simulink model "dadtetest"  (R2024a)
settings: Solver=VariableStepAuto  StartTime=0.0  StopTime=1  RelTol=1e-3
libraries: simulink x1
settings Model: Creator=wsl  LastModifiedBy=wsl

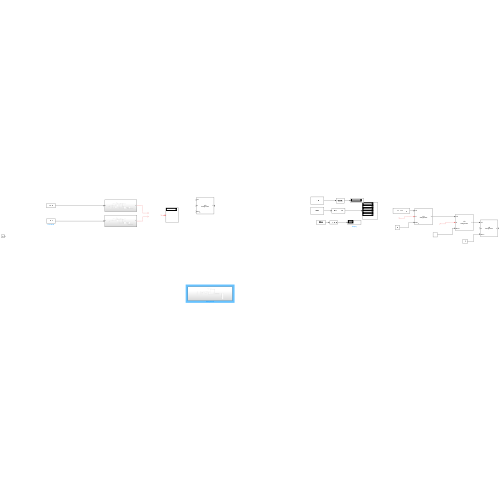
[thumbnail: Simulink's stored preview of the top-level diagram]
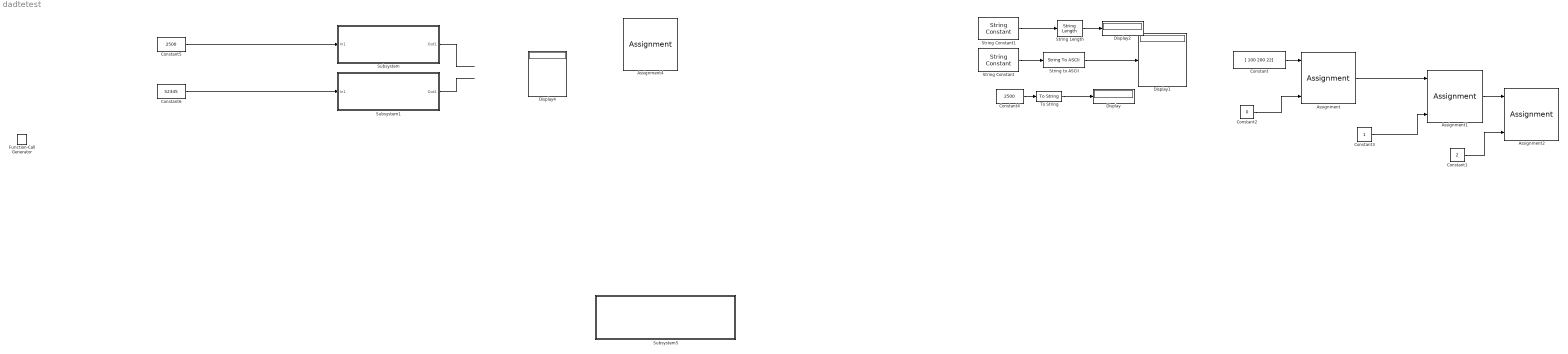
== system dadtetest ==
  Assignment : Assignment  IndexMode=Zero-based  DiagnosticForDimensions=Warning  IndexOptions=Index vector (port)  Indices=2  OutputSizes=1
  Assignment1 : Assignment  IndexMode=Zero-based  DiagnosticForDimensions=Warning  IndexOptions=Index vector (port)  Indices=2  OutputSizes=1
  Assignment2 : Assignment  IndexMode=Zero-based  DiagnosticForDimensions=Warning  IndexOptions=Index vector (port)  Indices=2  OutputSizes=1
  Assignment4 : Assignment  NumberOfDimensions=2  IndexMode=Zero-based  DiagnosticForDimensions=Warning  IndexOptions=Index vector (port),Index vector (dialog)  Indices=2,1  OutputSizes=1,1
  Constant : Constant  Value=[ 100 200 22]  OutDataTypeStr=single
  Constant1 : Constant  Value=2  OutDataTypeStr=uint8
  Constant2 : Constant  Value=0  OutDataTypeStr=uint8
  Constant3 : Constant  OutDataTypeStr=uint8
  Constant4 : Constant  Value=2500  OutDataTypeStr=uint16
  Constant5 : Constant  Value=2500  OutDataTypeStr=uint16
  Constant6 : Constant  Value=52345  OutDataTypeStr=uint16
  Display{,1..2,4} (4 alike) : Display
  Function-Call Generator : simulink/Ports & Subsystems/Function-Call Generator  sample_time=0.01  numberOfIterations=1  DisallowWideOutput=off
  String Constant : StringConstant  String='65535'
  String Constant1 : StringConstant  String='1234'
  String Length : StringLength  OutDataTypeStr=uint8
  String to ASCII : StringToASCII  OutputVectorSize=5
  Subsystem : Subsystem
  Subsystem1 : Subsystem
  Subsystem5 : Subsystem
  To String : ToString
  wires:
  Constant/1 -> Assignment/1
  ? -> Assignment/2
  Constant2/1 -> Assignment/3
  Assignment/1 -> Assignment1/1
  ? -> Assignment1/2
  Constant3/1 -> Assignment1/3
  Assignment1/1 -> Assignment2/1
  Constant1/1 -> Assignment2/3
  Constant4/1 -> To String/1
  To String/1 -> Display/1
  String to ASCII/1 -> Display1/1
  String Constant/1 -> String to ASCII/1
  String Length/1 -> Display2/1
  String Constant1/1 -> String Length/1
  Constant5/1 -> Subsystem/1(In1)
  Constant6/1 -> Subsystem1/1(In1)
  Subsystem/1(Out1) -> ?
  Subsystem1/1(Out1) -> ?
  ? -> Display4/1

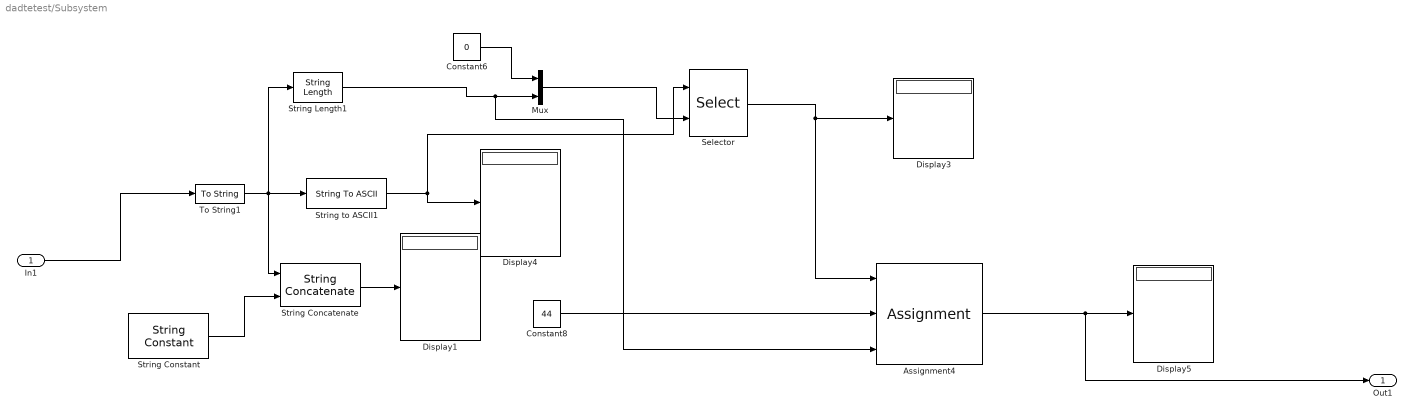
== system dadtetest/Subsystem ==
  In1 : Inport
  Assignment4 : Assignment  IndexMode=Zero-based  DiagnosticForDimensions=Warning  IndexOptions=Index vector (port)  Indices=2  OutputSizes=1
  Constant6 : Constant  Value=0  OutDataTypeStr=uint8
  Constant8 : Constant  Value=44  OutDataTypeStr=uint8
  Display{1,3..5} (4 alike) : Display
  Mux : Mux  Inputs=2
  Selector : Selector  IndexMode=Zero-based  InputPortWidth=6  IndexOptions=Starting and ending indices (port)  Indices=[1 3]  OutputSizes=1
  String Concatenate : StringConcatenate
  String Constant : StringConstant  String="\",\""
  String Length1 : StringLength  OutDataTypeStr=uint8
  String to ASCII1 : StringToASCII  OutputVectorSize=6
  To String1 : ToString
  Out1 : Outport
  wires:
  In1/1 -> To String1/1
  String Length1/1 -> Assignment4/3, Mux/2
  Constant6/1 -> Mux/1
  Constant8/1 -> Assignment4/2
  String to ASCII1/1 -> Selector/1, Display4/1
  Selector/1 -> Assignment4/1, Display3/1
  Mux/1 -> Selector/2
  Assignment4/1 -> Out1/1, Display5/1
  To String1/1 -> String Concatenate/1, String Length1/1, String to ASCII1/1
  String Constant/1 -> String Concatenate/2
  String Concatenate/1 -> Display1/1

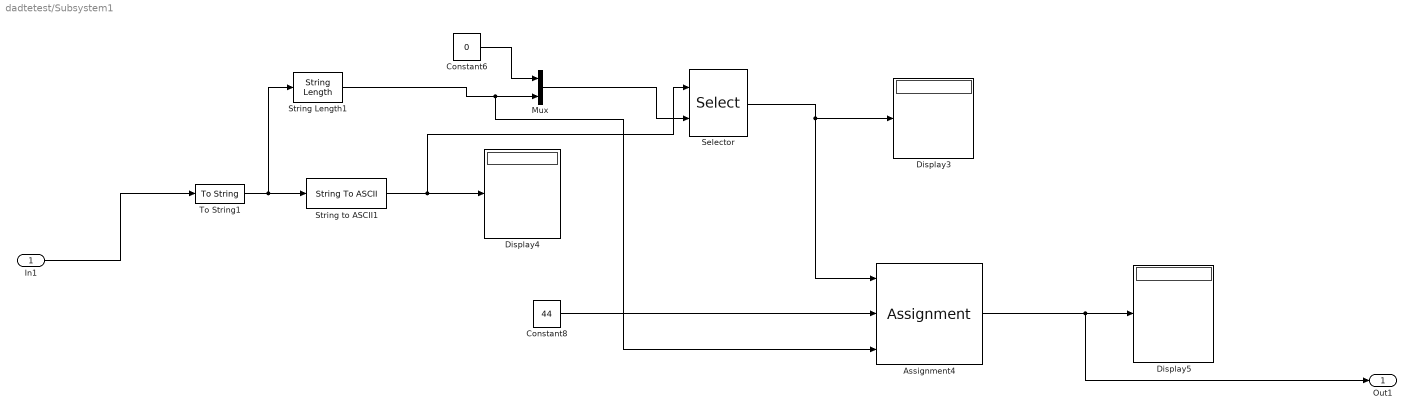
== system dadtetest/Subsystem1 ==
  In1 : Inport
  Assignment4 : Assignment  IndexMode=Zero-based  DiagnosticForDimensions=Warning  IndexOptions=Index vector (port)  Indices=2  OutputSizes=1
  Constant6 : Constant  Value=0  OutDataTypeStr=uint8
  Constant8 : Constant  Value=44  OutDataTypeStr=uint8
  Display3 : Display
  Display4 : Display
  Display5 : Display
  Mux : Mux  Inputs=2
  Selector : Selector  IndexMode=Zero-based  InputPortWidth=6  IndexOptions=Starting and ending indices (port)  Indices=[1 3]  OutputSizes=1
  String Length1 : StringLength  OutDataTypeStr=uint8
  String to ASCII1 : StringToASCII  OutputVectorSize=6
  To String1 : ToString
  Out1 : Outport
  wires:
  In1/1 -> To String1/1
  String Length1/1 -> Assignment4/3, Mux/2
  Constant6/1 -> Mux/1
  Constant8/1 -> Assignment4/2
  String to ASCII1/1 -> Selector/1, Display4/1
  Selector/1 -> Assignment4/1, Display3/1
  Mux/1 -> Selector/2
  Assignment4/1 -> Out1/1, Display5/1
  To String1/1 -> String Length1/1, String to ASCII1/1

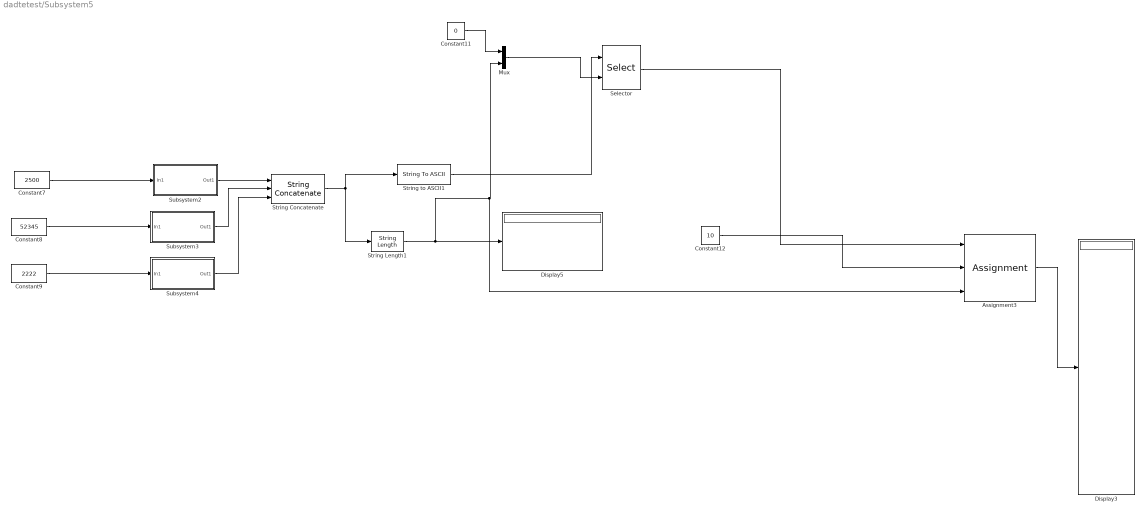
== system dadtetest/Subsystem5 ==
  Assignment3 : Assignment  IndexMode=Zero-based  DiagnosticForDimensions=Warning  IndexOptions=Index vector (port)  Indices=2  OutputSizes=1
  Constant11 : Constant  Value=0  OutDataTypeStr=uint8
  Constant12 : Constant  Value=10  OutDataTypeStr=uint8
  Constant7 : Constant  Value=2500  OutDataTypeStr=uint16
  Constant8 : Constant  Value=52345  OutDataTypeStr=uint16
  Constant9 : Constant  Value=2222  OutDataTypeStr=uint16
  Display3 : Display
  Display5 : Display
  Mux : Mux  Inputs=2
  Selector : Selector  IndexMode=Zero-based  InputPortWidth=32  IndexOptions=Starting and ending indices (port)  Indices=[1 3]  OutputSizes=1
  String Concatenate : StringConcatenate  Inputs=3
  String Length1 : StringLength  OutDataTypeStr=uint8
  String to ASCII1 : StringToASCII  OutputVectorSize=32
  Subsystem2 : Subsystem
  Subsystem3 : Subsystem
  Subsystem4 : Subsystem
  wires:
  Constant8/1 -> Subsystem3/1(In1)
  Subsystem4/1(Out1) -> String Concatenate/3
  Constant7/1 -> Subsystem2/1(In1)
  Constant9/1 -> Subsystem4/1(In1)
  Constant12/1 -> Assignment3/2
  String Length1/1 -> Assignment3/3, Mux/2, Display5/1
  Subsystem3/1(Out1) -> String Concatenate/2
  Mux/1 -> Selector/2
  Subsystem2/1(Out1) -> String Concatenate/1
  Constant11/1 -> Mux/1
  String to ASCII1/1 -> Selector/1
  String Concatenate/1 -> String Length1/1, String to ASCII1/1
  Assignment3/1 -> Display3/1
  Selector/1 -> Assignment3/1

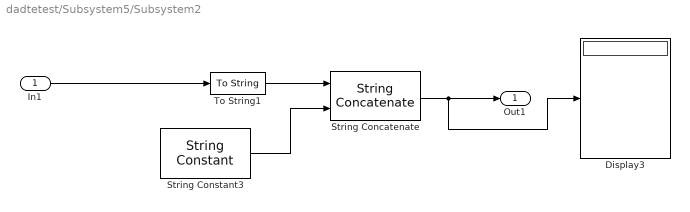
== system dadtetest/Subsystem5/Subsystem2 ==
  In1 : Inport
  Display3 : Display
  String Concatenate : StringConcatenate
  String Constant3 : StringConstant  String="\",\""
  To String1 : ToString
  Out1 : Outport
  wires:
  To String1/1 -> String Concatenate/1
  String Concatenate/1 -> Out1/1, Display3/1
  In1/1 -> To String1/1
  String Constant3/1 -> String Concatenate/2

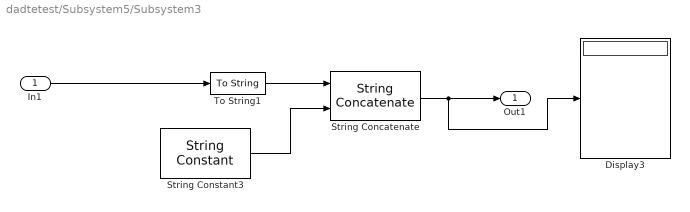
== system dadtetest/Subsystem5/Subsystem3 ==
  In1 : Inport
  Display3 : Display
  String Concatenate : StringConcatenate
  String Constant3 : StringConstant  String="\",\""
  To String1 : ToString
  Out1 : Outport
  wires:
  To String1/1 -> String Concatenate/1
  String Concatenate/1 -> Out1/1, Display3/1
  In1/1 -> To String1/1
  String Constant3/1 -> String Concatenate/2

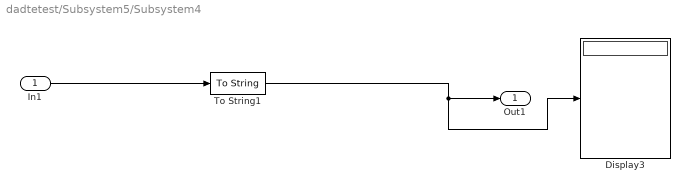
== system dadtetest/Subsystem5/Subsystem4 ==
  In1 : Inport
  Display3 : Display
  To String1 : ToString
  Out1 : Outport
  wires:
  To String1/1 -> Out1/1, Display3/1
  In1/1 -> To String1/1
